simulink model "rocket_airbrakes"  (R2026a)
settings: Solver=VariableStepAuto  StopTime=20
settings Model: Creator=eqtran103  LastModifiedBy=eqtran103

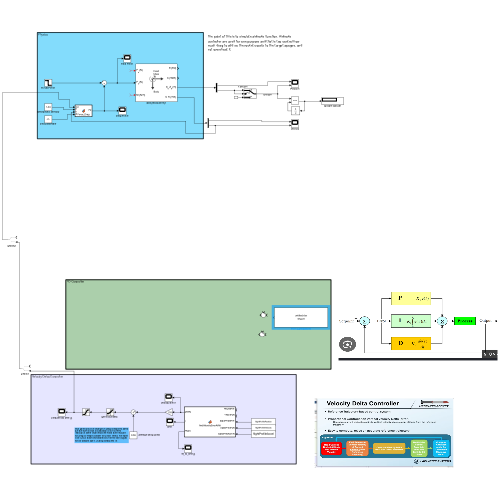
[thumbnail: Simulink's stored preview of the top-level diagram]
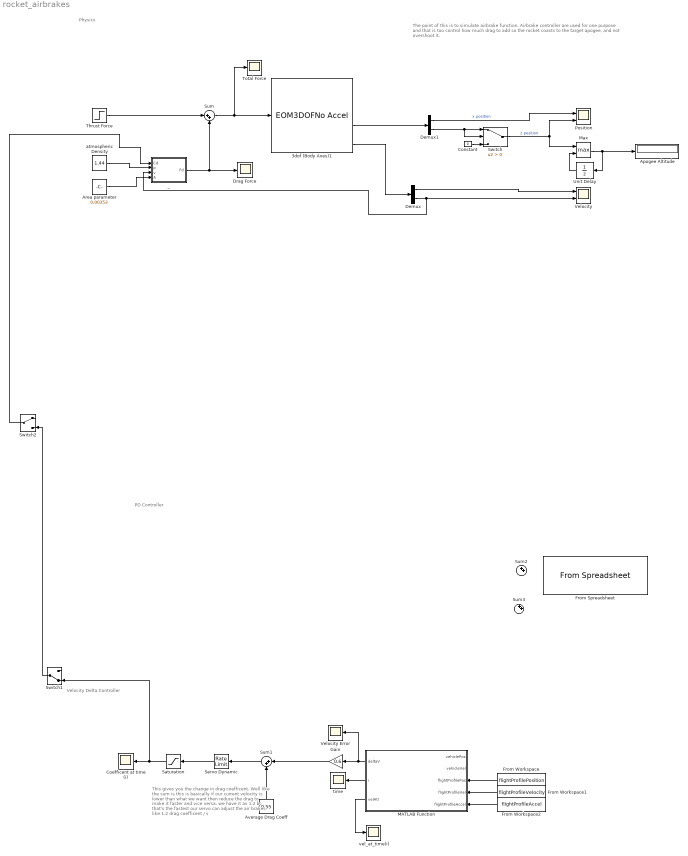
== system rocket_airbrakes ==
  note: This gives you the change in drag coefficent. Well like the sum is this is basically if our current velocity is lower than what we want then reduce the drag to make it faster and vice versa. we have it as 1.2 bc that's the fastest our servo can adjust the air brakes like 1.2 drag coefficent / s
  note: The point of this is to simulate airbrake function. Airbrake controller are used for one purpose and that is too control how much drag to add so the rocket coasts to the target apogee, and not overshoot it.
  note: Velocity Delta Controller
  note: Physics
  note: PD Controller
  3dof (Body Axes)1 : EOM3DOFNoAccel  v_ini=0  g=-9.81
  Apogee Altitude : Display
  Area parameter : Constant  Value=0.00353
  Average Drag Coeff : Constant  Value=0.55
  Coefficent at time (i) : Scope
      settings: DataLoggingVariableName=ScopeData7
  Constant : Constant  Value=0
  Demux : Demux  Outputs=2
  Demux1 : Demux  Outputs=2
  Drag Force : Scope
      settings: DataLoggingVariableName=ScopeData3
  From Workspace : FromWorkspace  VariableName=flightProfilePosition
  From Workspace1 : FromWorkspace  VariableName=flightProfileVelocity
  From Workspace2 : FromWorkspace  VariableName=flightProfileAccel
  From Spreadsheet : FromSpreadsheet
  Gain : Gain  Gain=0.6
  MATLAB Function : MATLAB Function  TreatAsAtomicUnit=on
  Max : MinMax  Function=max  Inputs=2
  Position : Scope  NumInputPorts=2
      settings: ActiveDisplayYMinimum=-25.950121313754732  ActiveDisplayYMaximum=233.55109182379266
  Saturation : Saturate  UpperLimit=0.7  LowerLimit=0.4  LinearizeAsGain=off
  "Servo Dynamic " : RateLimiter  RisingSlewLimit=1.2  FallingSlewLimit=-1.2  SampleTimeMode=inherited
  Sum : Sum  Inputs=|++
  Sum1 : Sum  Inputs=|++
  Sum2 : Sum  Inputs=++|
  Sum3 : Sum  Inputs=++|
  Switch : Switch  Criteria=u2 > Threshold  SaturateOnIntegerOverflow=off  InputSameDT=off
  Switch1 : ManualSwitch  CurrentSetting=0
  Switch2 : ManualSwitch
  Thrust Force : Step  Time=1.8  InitialValue=44  FinalValue=0  SampleTime=0
  Total Force : Scope
      settings: ActiveDisplayYMinimum=-118.76035736515115  ActiveDisplayYMaximum=62.084484151683455  DataLoggingVariableName=ScopeData2
  Unit Delay : UnitDelay  InitialCondition=-inf  SampleTime=-1
  Velocity : Scope  NumInputPorts=2
      settings: ActiveDisplayYMinimum=-369.03699440182197  ActiveDisplayYMaximum=106.92774455695476
  Velocity Error : Scope
      settings: DataLoggingVariableName=ScopeData6
  _ : MATLAB Function  TreatAsAtomicUnit=on
  atmospheric Density : Constant  Value=1.44
  time : Scope
      settings: DataLoggingVariableName=ScopeData5
  vel_at_time(i) : Scope
      settings: DataLoggingVariableName=ScopeData4
  wires:
  Demux1/2 -> Switch/1, Switch/2
  Constant/1 -> Switch/3
  Demux1/1 -> Position/1  "x position"
  Switch/1 -> Max/1, Position/2  "z position"
  Max/1 -> Unit Delay/1, Apogee Altitude/1
  Unit Delay/1 -> Max/2
  Demux/1 -> Velocity/1
  Switch2/1 -> _/1(Cd)
  ? -> 3dof (Body Axes)1/3
  atmospheric Density/1 -> _/2(p)
  3dof (Body Axes)1/4 -> Demux/1
  Sum/1 -> Total Force/1, 3dof (Body Axes)1/2
  Thrust Force/1 -> Sum/1
  _/1(Fd) -> Drag Force/1, Sum/2
  Area parameter/1 -> _/4(A)
  3dof (Body Axes)1/3 -> Demux1/1
  Demux/2 -> _/3(v), Velocity/2
  ? -> 3dof (Body Axes)1/1
  MATLAB Function/3(velAtI) -> vel_at_time(i)/1
  MATLAB Function/2(i) -> time/1
  MATLAB Function/1(deltaV) -> Velocity Error/1, Gain/1
  From Workspace2/1 -> MATLAB Function/5(flightProfileAccel)
  From Workspace1/1 -> MATLAB Function/4(flightProfileVel)
  From Workspace/1 -> MATLAB Function/3(flightProfilePos)
  Average Drag Coeff/1 -> Sum1/2
  Gain/1 -> Sum1/1
  Sum1/1 -> "Servo Dynamic "/1
  "Servo Dynamic "/1 -> Saturation/1
  Saturation/1 -> Switch1/2, Coefficent at time (i)/1
  Switch1/1 -> Switch2/2

== matlab function rocket_airbrakes/MATLAB Function ==
  data: vehiclePos input; deltaV output; i output; velAtI output; vehicleVel input; flightProfilePos input; flightProfileVel input; flightProfileAccel input
% Positive Numbers mean we are going faster and negative means slower
function [deltaV, i, velAtI] = findVelocityErrorAtAlt(vehiclePos, vehicleVel, flightProfilePos, flightProfileVel, flightProfileAccel)

n = size(flightProfilePos, 1);
lo = 1;
hi = n;
i = n;  % fallback if vehiclePos exceeds every entry

% binary search for first index where flightProfilePos(idx) >= vehiclePos
while lo <= hi
    mid = floor((lo + hi) / 2);
    if flightProfilePos(mid) >= vehiclePos
        i = mid;
        hi = mid - 1;
    else
        lo = mid + 1;
    end
end

if i == 1
    % vehiclePos at or below the very first sample, nothing to interpolate against
    velAtI = flightProfileVel(1);
else
    pos0 = flightProfilePos(i-1); pos1 = flightProfilePos(i);
    vel0 = flightProfileVel(i-1); vel1 = flightProfileVel(i);

    h = pos1 - pos0;
    t = (vehiclePos - pos0) / h;   % fraction across the gap, 0 to 1

    % Hermite interpolation: matches both value and slope (dv/dpos)
    % at each end, using acceleration from the logged reference profile.
    % dv/dpos = (dv/dt)/(dpos/dt) = acceleration/velocity (chain rule)
    slope0 = flightProfileAccel(i-1) / vel0;
    slope1 = flightProfileAccel(i)   / vel1;

    h00 = 2*t^3 - 3*t^2 + 1;
    h10 = t^3 - 2*t^2 + t;
    h01 = -2*t^3 + 3*t^2;
    h11 = t^3 - t^2;

    velAtI = h00*vel0 + h10*h*slope0 + h01*vel1 + h11*h*slope1;
end

deltaV = vehicleVel - velAtI;

end

== matlab function rocket_airbrakes/_ ==
  data: Cd input; Fd output; p input; v input; A input
% getting the drag force
function Fd = Force_Drag(Cd,p,v,A)

Fd = - 1/2 * Cd * p * v^2 * A;

end
% Fd =  Drag Force
% Cd = Drag Coefficent
% p = atmospheric Density
% v = current velocity
% A = Rocket Reference Area
